simulink model "FOC_Simulate"  (R2023a)
settings: Solver=FixedStepDiscrete  StartTime=0.0  StopTime=2  FixedStep=1e-6  RelTol=1e-3
values from neighbouring files (symbols this model uses):
  amplitude_voltage = 12    [PMSM_default.m]
  pair_num = 4    [PMSM_default.m]
  speed_pid_d = 0.0    (= 0)    [PMSM_default.m]
  speed_pid_i = 10.0    (= 10)    [PMSM_default.m]
  speed_pid_integ_limit = 50.0    (= 50)    [PMSM_default.m]
  speed_pid_out_limit = 200.0    (= 200)    [PMSM_default.m]
  speed_pid_p = 50.0    (= 50)    [PMSM_default.m]
  svpwm_period = 1/1000    (= 0.001)    [PMSM_default.m]
  torque_Id_integ_limit = 10.0    (= 10)    [PMSM_default.m]
  torque_Id_out_limit = 100.0    (= 100)    [PMSM_default.m]
  torque_Id_pid_i = 5.0    (= 5)    [PMSM_default.m]
  torque_Id_pid_p = 75.0    (= 75)    [PMSM_default.m]
  torque_Iq_integ_limit = 20.0    (= 20)    [PMSM_default.m]
  torque_Iq_out_limit = 100.0    (= 100)    [PMSM_default.m]
  torque_Iq_pid_d = 0.0    (= 0)    [PMSM_default.m]
  torque_Iq_pid_i = 1.0    (= 1)    [PMSM_default.m]
  torque_Iq_pid_p = 1.0    (= 1)    [PMSM_default.m]
libraries: slpidlib x4, simulink x2, spsDCVoltageSourceLib x1, spsPermanentMagnetSynchronousMachineLib x1, spsTwoLevelConverterLib x1, sps_lib x1
settings Model: Creator=72698  LastModifiedBy=72698
settings SolverCC: AutoInsertRateTranBlk=on

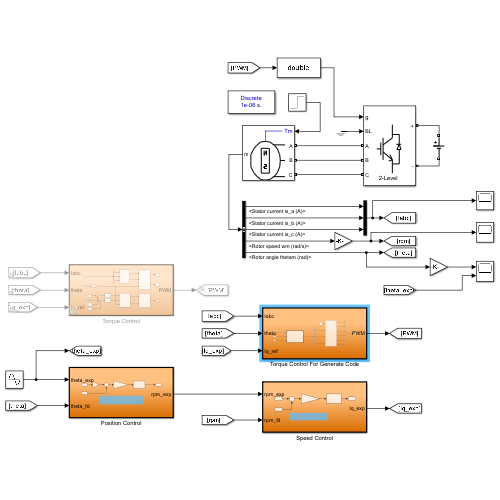
[thumbnail: Simulink's stored preview of the top-level diagram]
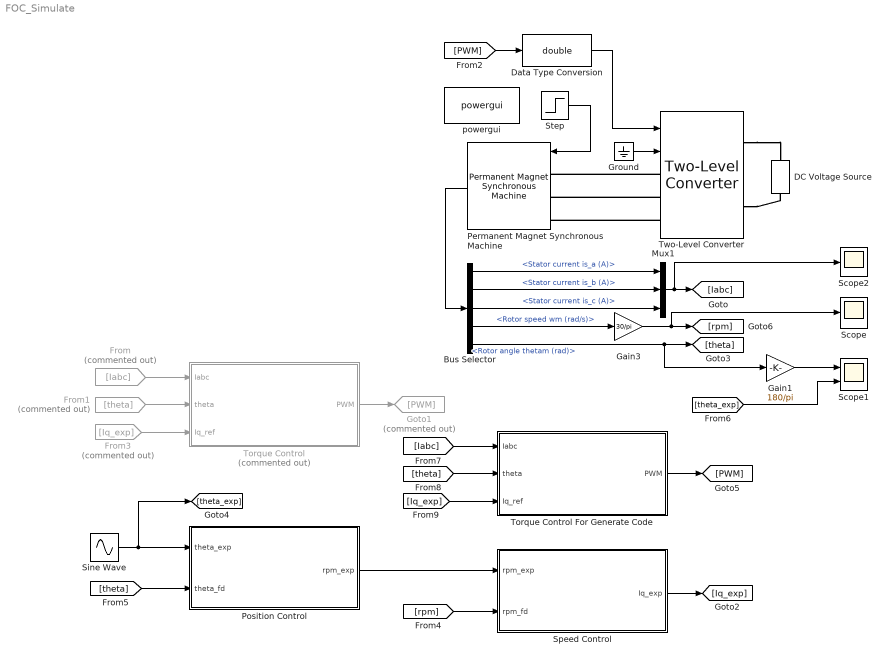
== system FOC_Simulate ==
  Bus Selector : BusSelector  OutputSignals=Stator current is_a (A),Stator current is_b (A),Stator current is_c (A),Rotor speed wm (rad/s),Rotor angle thetam (rad)
  DC Voltage Source : spsDCVoltageSourceLib/DC Voltage Source  Amplitude=amplitude_voltage  Measurements=None
  Data Type Conversion : DataTypeConversion  OutDataTypeStr=double  SaturateOnIntegerOverflow=off  RndMeth=Floor
  From : From  Commented=on  GotoTag=Iabc
  From1 : From  Commented=on  GotoTag=theta
  From3 : From  Commented=on  GotoTag=Iq_exp
  Gain1 : Gain  Gain=180/pi
  Gain3 : Gain  Gain=30/pi
  Goto1 : Goto  Commented=on  GotoTag=PWM
  Ground : Ground
  Mux1 : Mux  Inputs=3
  Permanent Magnet Synchronous Machine : spsPermanentMagnetSynchronousMachineLib/Permanent Magnet Synchronous Machine  NbPhases=3  FluxDistribution=Sinusoidal  RotorType=Round  MechanicalLoad=Torque Tm  PresetModel=No  ShowDetailedParameters=on  MeasurementBus=off  Resistance=0.0485  Inductance=8.5e-3  dqInductances=[8.5e-3,8.5e-3]  La=0.000395  MachineConstant=Flux linkage established by magnets (V.s)  Flux=0.1194  VoltageCst=86.6271  TorqueCst=0.7164  Flat=120  Mechanical=[0.0027 0.0004924 pair_num 0]  PolePairs=4  InitialConditions=[0,0, 0,0]  InitialConditions5ph=[0 0 0 0 0 0]  RefAngle=Aligned with phase A axis (original Park)  IterativeDiscreteModel=Trapezoidal non iterative  TsBlock=-1  TsPowergui=0
  Position Control : Subsystem  TreatAsAtomicUnit=on
  Scope : Scope
  Scope1 : Scope  NumInputPorts=2
  Scope2 : Scope
  Sine Wave : Sin  Amplitude=100  Frequency=10  SampleTime=0
  Speed Control : Subsystem  TreatAsAtomicUnit=on
  Step : Step  Time=0.2  After=10  SampleTime=0
  Torque Control : Subsystem  Commented=on  TreatAsAtomicUnit=on
  Torque Control For Generate Code : Subsystem  TreatAsAtomicUnit=on
  Two-Level Converter : spsTwoLevelConverterLib/Two-Level Converter  ModelType=Switching devices  Ron=1e-3  Rs=1e6  Cs=inf  Vforward=[0,0]  Ron_Diode=1e-3  Rs_Diode=1e6  Cs_Diode=inf  Vf_Diode=1e-3  Rs_CurrentSource=inf  Ron_ACsource=1e-3
      settings: LibrarySourceBlock=sps_lib/Power Electronics/Two-Level Converter
  powergui : sps_lib/powergui  Priority=1  SimulationMode=Discrete  SampleTime=1e-6  frequency=60  Iterations=50  frequencyindice=0  Pbase=100e6  ErrMax=1e-4  UnitsV=kV  UnitsW=MW  buscounter=0  FunctionMessages=off  echomessages=off  EnableUseOfTLC=off  CurrentSourceSwitches=off  DisableSnubberDevices=off  DisableRonSwitches=off  DisableVfSwitches=off  DisplayEquations=off  AutomaticDiscreteSolvers=off  SolverType=Tustin/Backward Euler (TBE)  Interpol=off  ExternalGateDelay=off  methode=off  Ts=100  x0status=blocks  SPID=on  SwTol=0  HookPort=off  NonlinearTolerance=1e-4  nMaxIteration=100  ContinueOnMaxIteration=off  RestoreLinks=warning  ResistiveCurrentMeasurement=off  Frange=[0:2:500]  Ylog=off  Xlog=on  ShowGrid=off  save=off  variable=ZData  structure=0  ZoomFFT=off  StartTime=0.0  cycles=1  DisplayStyle=1  fundamental=60  FreqAxis=off  MaxFrequency=1000  frequencyindicesteady=1  RmsSteady=1  display=off
  wires:
  Ground/1 -> Two-Level Converter/2
  Step/1 -> Permanent Magnet Synchronous Machine/1
  Permanent Magnet Synchronous Machine/1 -> Bus Selector/1
  Data Type Conversion/1 -> Two-Level Converter/1
  Bus Selector/4 -> Gain3/1  "<Rotor speed wm (rad/s)>"
  Bus Selector/5 -> Gain1/1, [theta]  "<Rotor angle thetam (rad)>"
  Bus Selector/1 -> Mux1/1  "<Stator current is_a (A)>"
  Bus Selector/2 -> Mux1/2  "<Stator current is_b (A)>"
  Bus Selector/3 -> Mux1/3  "<Stator current is_c (A)>"
  Mux1/1 -> Scope2/1, [Iabc]
  Gain3/1 -> Scope/1, [rpm]
  [PWM] -> Data Type Conversion/1
  [rpm] -> Speed Control/2(rpm_fd)
  Speed Control/1(Iq_exp) -> [Iq_exp]
  Gain1/1 -> Scope1/1
  Position Control/1(rpm_exp) -> Speed Control/1(rpm_exp)
  [theta] -> Position Control/2(theta_fd)
  Sine Wave/1 -> [theta_exp], Position Control/1(theta_exp)
  [theta_exp] -> Scope1/2
  Torque Control For Generate Code/1(PWM) -> [PWM]
  [theta] -> Torque Control For Generate Code/2(theta)
  [Iabc] -> Torque Control For Generate Code/1(Iabc)
  [Iq_exp] -> Torque Control For Generate Code/3(Iq_ref)
  Torque Control/1(PWM) -> Goto1/1
  From1/1 -> Torque Control/2(theta)
  From/1 -> Torque Control/1(Iabc)
  From3/1 -> Torque Control/3(Iq_ref)
  connections:
  Two-Level Converter/LConn1 -- Permanent Magnet Synchronous Machine/LConn1
  Two-Level Converter/LConn2 -- Permanent Magnet Synchronous Machine/LConn2
  Two-Level Converter/LConn3 -- Permanent Magnet Synchronous Machine/LConn3
  Two-Level Converter/RConn1 -- DC Voltage Source/RConn1
  Two-Level Converter/RConn2 -- DC Voltage Source/LConn1

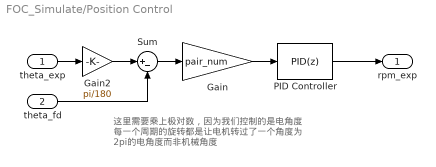
== system FOC_Simulate/Position Control ==
  note: 这里需要乘上极对数，因为我们控制的是电角度
      | 每一个周期的旋转都是让电机转过了一个角度为
      | 2pi的电角度而非机械角度
  theta_exp : Inport
  theta_fd : Inport  Port=2
  Gain : Gain  Gain=pair_num
  Gain2 : Gain  Gain=pi/180
  PID Controller : slpidlib/PID Controller  Controller=PID  Form=Parallel  TimeDomain=Discrete-time  UseExternalTs=off  SampleTime=-1  IntegratorMethod=Forward Euler  FilterMethod=Forward Euler  ControllerParametersSource=internal  P=95  I=0  UseKiTs=off  D=0  N=100  UseFilter=on  TunerSelectOption=Transfer Function Based (PID Tuner App)  InitialConditionSource=internal  InitialConditionForIntegrator=0  InitialConditionForFilter=0  DifferentiatorICPrevScaledInput=0  ExternalReset=none  TrackingMode=off  Kt=1  LimitOutput=on  SatLimitsSource=internal  UpperSaturationLimit=speed_pid_out_limit  LowerSaturationLimit=-speed_pid_out_limit  LinearizeAsGain=on  AntiWindupMode=none  Kb=1  LimitIntegrator=on  UpperIntegratorSaturationLimit=speed_pid_integ_limit  LowerIntegratorSaturationLimit=-speed_pid_integ_limit  POutMin=[]  POutMax=[]  IOutMin=[]  IOutMax=[]  DOutMin=[]  DOutMax=[]  NOutMin=[]  NOutMax=[]  SumOutMin=[]  SumOutMax=[]  SaturationOutMin=[]  SaturationOutMax=[]  PParamMin=[]  PParamMax=[]  IParamMin=[]  IParamMax=[]  DParamMin=[]  DParamMax=[]  NParamMin=[]  NParamMax=[]  KbParamMin=[]  KbParamMax=[]  KtParamMin=[]  KtParamMax=[]  KbOutMin=[]  KbOutMax=[]  KtOutMin=[]  KtOutMax=[]  IntegratorOutMin=[]  IntegratorOutMax=[]  FilterOutMin=[]  FilterOutMax=[]  SumI1OutMin=[]  SumI1OutMax=[]  SumI2OutMin=[]  SumI2OutMax=[]  SumI3OutMin=[]  SumI3OutMax=[]  SumI4OutMin=[]  SumI4OutMax=[]  SumDOutMin=[]  SumDOutMax=[]  DifferentiatorOutMin=[]  DifferentiatorOutMax=[]  FilterDiffOutCoefMin=[]  FilterDiffOutCoefMax=[]  ReciprocalOutMin=[]  ReciprocalOutMax=[]  SumDenOutMin=[]  SumDenOutMax=[]  SumNumOutMin=[]  SumNumOutMax=[]  DivideOutMin=[]  DivideOutMax=[]  UdiffTsProdOutMin=[]  UdiffTsProdOutMax=[]  NTsProdOutMin=[]  NTsProdOutMax=[]  UintegralTsProdOutMin=[]  UintegralTsProdOutMax=[]  UngainTsProdOutMin=[]  UngainTsProdOutMax=[]  ClampingZeroOutDataTypeStr=Inherit: Inherit via back propagation  ClampingZeroOutMin=[]  ClampingZeroOutMax=[]  FilterDenConstantOutDataTypeStr=Inherit: Inherit via back propagation  FilterDenConstantOutMin=[]  FilterDenConstantOutMax=[]  PCopyOutDataTypeStr=Inherit: Inherit via back propagation  PCopyOutMin=[]  PCopyOutMax=[]  NCopyOutDataTypeStr=Inherit: Inherit via back propagation  NCopyOutMin=[]  NCopyOutMax=[]  IntegratorContinuousStateAttributes=''  IntegratorStateMustResolveToSignalObject=off  IntegratorRTWStateStorageClass=Auto  FilterContinuousStateAttributes=''  FilterStateMustResolveToSignalObject=off  FilterRTWStateStorageClass=Auto  ParallelPVariant=InternalParameters  IdealPVariant=Disabled  IVariant=InternalParameters  DVariant=InternalParameters  IntegratorVariant=Discrete  SatVariant=Enabled  AWVariant=Passthrough  PCopyVariant=Disabled  TRVariant=Disabled  FdbkBlocksVariant=Forward  IdealPFdbkVariant=Disabled  SatFdbkVariant=Disabled  DerivativeFilterVariant=ForwardEulerFilter  NVariant=InternalParameters  NCopyVariant=Disabled  FilterICVariant=InternalICsFilter  IntegratorICVariant=InternalICs  ExternalResetVariant=Disabled  TRSumVariant=Passthrough  SumFdbkVariant=Disabled  SumVariant=Sum_PID  TsampFilterVariant=InternalTs  TsampNgainVariant=Passthrough  TsampIntegralVariant=Disabled_SignalSpec  ExternalSaturationOutDataTypeStr=Inherit: Same as second input
  Sum : Sum  Inputs=|+-
  rpm_exp : Outport
  wires:
  Gain/1 -> PID Controller/1
  Gain2/1 -> Sum/1
  theta_exp/1 -> Gain2/1
  Sum/1 -> Gain/1
  theta_fd/1 -> Sum/2
  PID Controller/1 -> rpm_exp/1

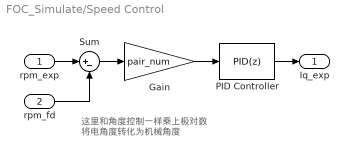
== system FOC_Simulate/Speed Control ==
  note: 这里和角度控制一样乘上极对数
      | 将电角度转化为机械角度
  rpm_exp : Inport
  rpm_fd : Inport  Port=2
  Gain : Gain  Gain=pair_num
  PID Controller : slpidlib/PID Controller  Controller=PID  Form=Parallel  TimeDomain=Discrete-time  UseExternalTs=off  SampleTime=-1  IntegratorMethod=Forward Euler  FilterMethod=Forward Euler  ControllerParametersSource=internal  P=speed_pid_p  I=speed_pid_i  UseKiTs=off  D=speed_pid_d  N=100  UseFilter=on  TunerSelectOption=Transfer Function Based (PID Tuner App)  InitialConditionSource=internal  InitialConditionForIntegrator=0  InitialConditionForFilter=0  DifferentiatorICPrevScaledInput=0  ExternalReset=none  TrackingMode=off  Kt=1  LimitOutput=on  SatLimitsSource=internal  UpperSaturationLimit=speed_pid_out_limit  LowerSaturationLimit=-speed_pid_out_limit  LinearizeAsGain=on  AntiWindupMode=none  Kb=1  LimitIntegrator=on  UpperIntegratorSaturationLimit=speed_pid_integ_limit  LowerIntegratorSaturationLimit=-speed_pid_integ_limit  POutMin=[]  POutMax=[]  IOutMin=[]  IOutMax=[]  DOutMin=[]  DOutMax=[]  NOutMin=[]  NOutMax=[]  SumOutMin=[]  SumOutMax=[]  SaturationOutMin=[]  SaturationOutMax=[]  PParamMin=[]  PParamMax=[]  IParamMin=[]  IParamMax=[]  DParamMin=[]  DParamMax=[]  NParamMin=[]  NParamMax=[]  KbParamMin=[]  KbParamMax=[]  KtParamMin=[]  KtParamMax=[]  KbOutMin=[]  KbOutMax=[]  KtOutMin=[]  KtOutMax=[]  IntegratorOutMin=[]  IntegratorOutMax=[]  FilterOutMin=[]  FilterOutMax=[]  SumI1OutMin=[]  SumI1OutMax=[]  SumI2OutMin=[]  SumI2OutMax=[]  SumI3OutMin=[]  SumI3OutMax=[]  SumI4OutMin=[]  SumI4OutMax=[]  SumDOutMin=[]  SumDOutMax=[]  DifferentiatorOutMin=[]  DifferentiatorOutMax=[]  FilterDiffOutCoefMin=[]  FilterDiffOutCoefMax=[]  ReciprocalOutMin=[]  ReciprocalOutMax=[]  SumDenOutMin=[]  SumDenOutMax=[]  SumNumOutMin=[]  SumNumOutMax=[]  DivideOutMin=[]  DivideOutMax=[]  UdiffTsProdOutMin=[]  UdiffTsProdOutMax=[]  NTsProdOutMin=[]  NTsProdOutMax=[]  UintegralTsProdOutMin=[]  UintegralTsProdOutMax=[]  UngainTsProdOutMin=[]  UngainTsProdOutMax=[]  ClampingZeroOutDataTypeStr=Inherit: Inherit via back propagation  ClampingZeroOutMin=[]  ClampingZeroOutMax=[]  FilterDenConstantOutDataTypeStr=Inherit: Inherit via back propagation  FilterDenConstantOutMin=[]  FilterDenConstantOutMax=[]  PCopyOutDataTypeStr=Inherit: Inherit via back propagation  PCopyOutMin=[]  PCopyOutMax=[]  NCopyOutDataTypeStr=Inherit: Inherit via back propagation  NCopyOutMin=[]  NCopyOutMax=[]  IntegratorContinuousStateAttributes=''  IntegratorStateMustResolveToSignalObject=off  IntegratorRTWStateStorageClass=Auto  FilterContinuousStateAttributes=''  FilterStateMustResolveToSignalObject=off  FilterRTWStateStorageClass=Auto  ParallelPVariant=InternalParameters  IdealPVariant=Disabled  IVariant=InternalParameters  DVariant=InternalParameters  IntegratorVariant=Discrete  SatVariant=Enabled  AWVariant=Passthrough  PCopyVariant=Disabled  TRVariant=Disabled  FdbkBlocksVariant=Forward  IdealPFdbkVariant=Disabled  SatFdbkVariant=Disabled  DerivativeFilterVariant=ForwardEulerFilter  NVariant=InternalParameters  NCopyVariant=Disabled  FilterICVariant=InternalICsFilter  IntegratorICVariant=InternalICs  ExternalResetVariant=Disabled  TRSumVariant=Passthrough  SumFdbkVariant=Disabled  SumVariant=Sum_PID  TsampFilterVariant=InternalTs  TsampNgainVariant=Passthrough  TsampIntegralVariant=Disabled_SignalSpec  ExternalSaturationOutDataTypeStr=Inherit: Same as second input
  Sum : Sum  Inputs=|+-
  Iq_exp : Outport
  wires:
  rpm_exp/1 -> Sum/1
  rpm_fd/1 -> Sum/2
  Sum/1 -> Gain/1
  PID Controller/1 -> Iq_exp/1
  Gain/1 -> PID Controller/1

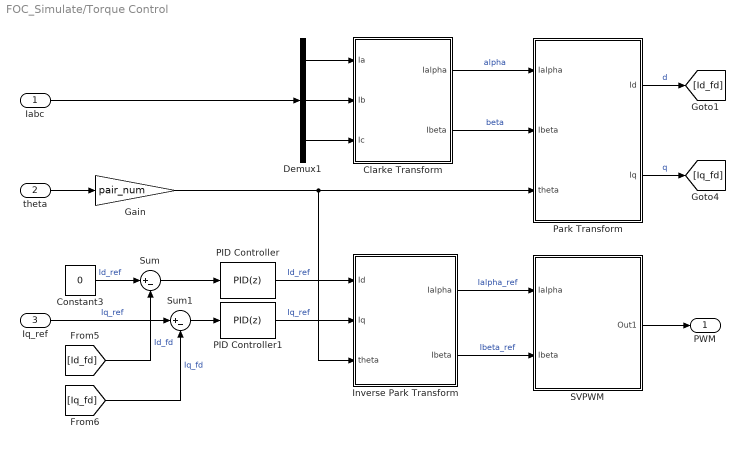
== system FOC_Simulate/Torque Control ==
  Iabc : Inport
  theta : Inport  Port=2
  Iq_ref : Inport  Port=3
  Clarke Transform : Subsystem  TreatAsAtomicUnit=on
  Constant3 : Constant  Value=0
  Demux1 : Demux  Outputs=3
  Gain : Gain  Gain=pair_num
  Inverse Park Transform : Subsystem  TreatAsAtomicUnit=on
  PID Controller : slpidlib/PID Controller  Controller=PID  Form=Parallel  TimeDomain=Discrete-time  UseExternalTs=off  SampleTime=-1  IntegratorMethod=Forward Euler  FilterMethod=Forward Euler  ControllerParametersSource=internal  P=torque_Id_pid_p  I=torque_Id_pid_i  UseKiTs=off  D=torque_Iq_pid_d  N=100  UseFilter=on  TunerSelectOption=Transfer Function Based (PID Tuner App)  InitialConditionSource=internal  InitialConditionForIntegrator=0  InitialConditionForFilter=0  DifferentiatorICPrevScaledInput=0  ExternalReset=none  TrackingMode=off  Kt=1  LimitOutput=on  SatLimitsSource=internal  UpperSaturationLimit=torque_Id_out_limit  LowerSaturationLimit=-torque_Id_out_limit  LinearizeAsGain=on  AntiWindupMode=none  Kb=1  LimitIntegrator=on  UpperIntegratorSaturationLimit=torque_Id_integ_limit  LowerIntegratorSaturationLimit=-torque_Id_integ_limit  POutMin=[]  POutMax=[]  IOutMin=[]  IOutMax=[]  DOutMin=[]  DOutMax=[]  NOutMin=[]  NOutMax=[]  SumOutMin=[]  SumOutMax=[]  SaturationOutMin=[]  SaturationOutMax=[]  PParamMin=[]  PParamMax=[]  IParamMin=[]  IParamMax=[]  DParamMin=[]  DParamMax=[]  NParamMin=[]  NParamMax=[]  KbParamMin=[]  KbParamMax=[]  KtParamMin=[]  KtParamMax=[]  KbOutMin=[]  KbOutMax=[]  KtOutMin=[]  KtOutMax=[]  IntegratorOutMin=[]  IntegratorOutMax=[]  FilterOutMin=[]  FilterOutMax=[]  SumI1OutMin=[]  SumI1OutMax=[]  SumI2OutMin=[]  SumI2OutMax=[]  SumI3OutMin=[]  SumI3OutMax=[]  SumI4OutMin=[]  SumI4OutMax=[]  SumDOutMin=[]  SumDOutMax=[]  DifferentiatorOutMin=[]  DifferentiatorOutMax=[]  FilterDiffOutCoefMin=[]  FilterDiffOutCoefMax=[]  ReciprocalOutMin=[]  ReciprocalOutMax=[]  SumDenOutMin=[]  SumDenOutMax=[]  SumNumOutMin=[]  SumNumOutMax=[]  DivideOutMin=[]  DivideOutMax=[]  UdiffTsProdOutMin=[]  UdiffTsProdOutMax=[]  NTsProdOutMin=[]  NTsProdOutMax=[]  UintegralTsProdOutMin=[]  UintegralTsProdOutMax=[]  UngainTsProdOutMin=[]  UngainTsProdOutMax=[]  ClampingZeroOutDataTypeStr=Inherit: Inherit via back propagation  ClampingZeroOutMin=[]  ClampingZeroOutMax=[]  FilterDenConstantOutDataTypeStr=Inherit: Inherit via back propagation  FilterDenConstantOutMin=[]  FilterDenConstantOutMax=[]  PCopyOutDataTypeStr=Inherit: Inherit via back propagation  PCopyOutMin=[]  PCopyOutMax=[]  NCopyOutDataTypeStr=Inherit: Inherit via back propagation  NCopyOutMin=[]  NCopyOutMax=[]  IntegratorContinuousStateAttributes=''  IntegratorStateMustResolveToSignalObject=off  IntegratorRTWStateStorageClass=Auto  FilterContinuousStateAttributes=''  FilterStateMustResolveToSignalObject=off  FilterRTWStateStorageClass=Auto  ParallelPVariant=InternalParameters  IdealPVariant=Disabled  IVariant=InternalParameters  DVariant=InternalParameters  IntegratorVariant=Discrete  SatVariant=Enabled  AWVariant=Passthrough  PCopyVariant=Disabled  TRVariant=Disabled  FdbkBlocksVariant=Forward  IdealPFdbkVariant=Disabled  SatFdbkVariant=Disabled  DerivativeFilterVariant=ForwardEulerFilter  NVariant=InternalParameters  NCopyVariant=Disabled  FilterICVariant=InternalICsFilter  IntegratorICVariant=InternalICs  ExternalResetVariant=Disabled  TRSumVariant=Passthrough  SumFdbkVariant=Disabled  SumVariant=Sum_PID  TsampFilterVariant=InternalTs  TsampNgainVariant=Passthrough  TsampIntegralVariant=Disabled_SignalSpec  ExternalSaturationOutDataTypeStr=Inherit: Same as second input
  PID Controller1 : slpidlib/PID Controller  Controller=PID  Form=Parallel  TimeDomain=Discrete-time  UseExternalTs=off  SampleTime=-1  IntegratorMethod=Forward Euler  FilterMethod=Forward Euler  ControllerParametersSource=internal  P=torque_Iq_pid_p  I=torque_Iq_pid_i  UseKiTs=off  D=torque_Iq_pid_d  N=100  UseFilter=on  TunerSelectOption=Transfer Function Based (PID Tuner App)  InitialConditionSource=internal  InitialConditionForIntegrator=0  InitialConditionForFilter=0  DifferentiatorICPrevScaledInput=0  ExternalReset=none  TrackingMode=off  Kt=1  LimitOutput=on  SatLimitsSource=internal  UpperSaturationLimit=torque_Iq_out_limit  LowerSaturationLimit=-torque_Iq_out_limit  LinearizeAsGain=on  AntiWindupMode=none  Kb=1  LimitIntegrator=on  UpperIntegratorSaturationLimit=torque_Iq_integ_limit  LowerIntegratorSaturationLimit=-torque_Iq_integ_limit  POutMin=[]  POutMax=[]  IOutMin=[]  IOutMax=[]  DOutMin=[]  DOutMax=[]  NOutMin=[]  NOutMax=[]  SumOutMin=[]  SumOutMax=[]  SaturationOutMin=[]  SaturationOutMax=[]  PParamMin=[]  PParamMax=[]  IParamMin=[]  IParamMax=[]  DParamMin=[]  DParamMax=[]  NParamMin=[]  NParamMax=[]  KbParamMin=[]  KbParamMax=[]  KtParamMin=[]  KtParamMax=[]  KbOutMin=[]  KbOutMax=[]  KtOutMin=[]  KtOutMax=[]  IntegratorOutMin=[]  IntegratorOutMax=[]  FilterOutMin=[]  FilterOutMax=[]  SumI1OutMin=[]  SumI1OutMax=[]  SumI2OutMin=[]  SumI2OutMax=[]  SumI3OutMin=[]  SumI3OutMax=[]  SumI4OutMin=[]  SumI4OutMax=[]  SumDOutMin=[]  SumDOutMax=[]  DifferentiatorOutMin=[]  DifferentiatorOutMax=[]  FilterDiffOutCoefMin=[]  FilterDiffOutCoefMax=[]  ReciprocalOutMin=[]  ReciprocalOutMax=[]  SumDenOutMin=[]  SumDenOutMax=[]  SumNumOutMin=[]  SumNumOutMax=[]  DivideOutMin=[]  DivideOutMax=[]  UdiffTsProdOutMin=[]  UdiffTsProdOutMax=[]  NTsProdOutMin=[]  NTsProdOutMax=[]  UintegralTsProdOutMin=[]  UintegralTsProdOutMax=[]  UngainTsProdOutMin=[]  UngainTsProdOutMax=[]  ClampingZeroOutDataTypeStr=Inherit: Inherit via back propagation  ClampingZeroOutMin=[]  ClampingZeroOutMax=[]  FilterDenConstantOutDataTypeStr=Inherit: Inherit via back propagation  FilterDenConstantOutMin=[]  FilterDenConstantOutMax=[]  PCopyOutDataTypeStr=Inherit: Inherit via back propagation  PCopyOutMin=[]  PCopyOutMax=[]  NCopyOutDataTypeStr=Inherit: Inherit via back propagation  NCopyOutMin=[]  NCopyOutMax=[]  IntegratorContinuousStateAttributes=''  IntegratorStateMustResolveToSignalObject=off  IntegratorRTWStateStorageClass=Auto  FilterContinuousStateAttributes=''  FilterStateMustResolveToSignalObject=off  FilterRTWStateStorageClass=Auto  ParallelPVariant=InternalParameters  IdealPVariant=Disabled  IVariant=InternalParameters  DVariant=InternalParameters  IntegratorVariant=Discrete  SatVariant=Enabled  AWVariant=Passthrough  PCopyVariant=Disabled  TRVariant=Disabled  FdbkBlocksVariant=Forward  IdealPFdbkVariant=Disabled  SatFdbkVariant=Disabled  DerivativeFilterVariant=ForwardEulerFilter  NVariant=InternalParameters  NCopyVariant=Disabled  FilterICVariant=InternalICsFilter  IntegratorICVariant=InternalICs  ExternalResetVariant=Disabled  TRSumVariant=Passthrough  SumFdbkVariant=Disabled  SumVariant=Sum_PID  TsampFilterVariant=InternalTs  TsampNgainVariant=Passthrough  TsampIntegralVariant=Disabled_SignalSpec  ExternalSaturationOutDataTypeStr=Inherit: Same as second input
  Park Transform : Subsystem  TreatAsAtomicUnit=on
  SVPWM : Subsystem  TreatAsAtomicUnit=on
  Sum : Sum  Inputs=|+-
  Sum1 : Sum  Inputs=|+-
  PWM : Outport
  wires:
  Park Transform/2(Iq) -> [Iq_fd]  "q"
  Iq_ref/1 -> Sum1/1  "Iq_ref"
  [Iq_fd] -> Sum1/2  "Iq_fd"
  [Id_fd] -> Sum/2  "Id_fd"
  Demux1/2 -> Clarke Transform/2(Ib)
  Clarke Transform/1(Ialpha) -> Park Transform/1(Ialpha)  "alpha"
  PID Controller1/1 -> Inverse Park Transform/2(Iq)  "Iq_ref"
  theta/1 -> Gain/1
  Inverse Park Transform/1(Ialpha) -> SVPWM/1(Ialpha)  "Ialpha_ref"
  SVPWM/1(Out1) -> PWM/1
  Inverse Park Transform/2(Ibeta) -> SVPWM/2(Ibeta)  "Ibeta_ref"
  Demux1/1 -> Clarke Transform/1(Ia)
  Demux1/3 -> Clarke Transform/3(Ic)
  PID Controller/1 -> Inverse Park Transform/1(Id)  "Id_ref"
  Sum1/1 -> PID Controller1/1
  Clarke Transform/2(Ibeta) -> Park Transform/2(Ibeta)  "beta"
  Park Transform/1(Id) -> [Id_fd]  "d"
  Sum/1 -> PID Controller/1
  Constant3/1 -> Sum/1  "Id_ref"
  Iabc/1 -> Demux1/1
  Gain/1 -> Park Transform/3(theta), Inverse Park Transform/3(theta)

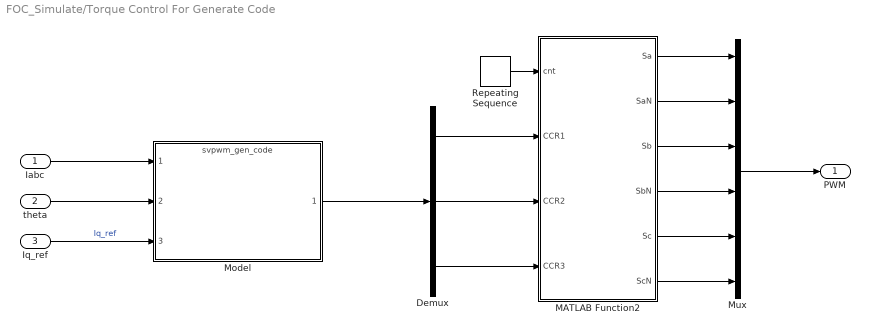
== system FOC_Simulate/Torque Control For Generate Code ==
  Iabc : Inport
  theta : Inport  Port=2
  Iq_ref : Inport  Port=3
  Demux : Demux  Outputs=3
  MATLAB Function2 : MATLAB Function  TreatAsAtomicUnit=on
  Model : ModelReference  ModelNameDialog=svpwm_gen_code.slx  SimulationMode=Normal  ModelReferenceVersion=1.1
  Mux : Mux  Inputs=6
  Repeating Sequence : simulink/Sources/Repeating Sequence  rep_seq_t=[0 svpwm_period/2 svpwm_period]  rep_seq_y=[0 svpwm_period/2 0]
  PWM : Outport
  wires:
  MATLAB Function2/4(SbN) -> Mux/4
  Repeating Sequence/1 -> MATLAB Function2/1(cnt)
  MATLAB Function2/5(Sc) -> Mux/5
  MATLAB Function2/6(ScN) -> Mux/6
  MATLAB Function2/3(Sb) -> Mux/3
  MATLAB Function2/1(Sa) -> Mux/1
  Demux/3 -> MATLAB Function2/4(CCR3)
  Demux/2 -> MATLAB Function2/3(CCR2)
  Demux/1 -> MATLAB Function2/2(CCR1)
  MATLAB Function2/2(SaN) -> Mux/2
  Iabc/1 -> Model/1
  theta/1 -> Model/2
  Iq_ref/1 -> Model/3  "Iq_ref"
  Model/1 -> Demux/1
  Mux/1 -> PWM/1

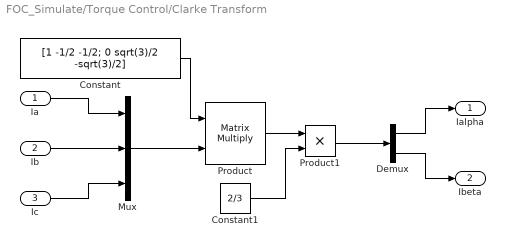
== system FOC_Simulate/Torque Control/Clarke Transform ==
  Ia : Inport
  Ib : Inport  Port=2
  Ic : Inport  Port=3
  Constant : Constant  Value=[1 -1/2 -1/2; 0 sqrt(3)/2 -sqrt(3)/2]
  Constant1 : Constant  Value=2/3
  Demux : Demux  Outputs=2
  Mux : Mux  Inputs=3
  Product : Product  Multiplication=Matrix(*)
  Product1 : Product
  Ialpha : Outport
  Ibeta : Outport  Port=2
  wires:
  Ib/1 -> Mux/2
  Ia/1 -> Mux/1
  Ic/1 -> Mux/3
  Mux/1 -> Product/2
  Constant/1 -> Product/1
  Demux/1 -> Ialpha/1
  Demux/2 -> Ibeta/1
  Product/1 -> Product1/1
  Product1/1 -> Demux/1
  Constant1/1 -> Product1/2

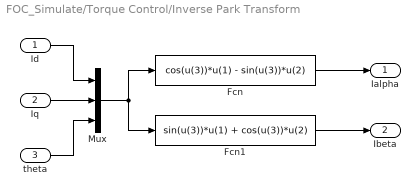
== system FOC_Simulate/Torque Control/Inverse Park Transform ==
  Id : Inport
  Iq : Inport  Port=2
  theta : Inport  Port=3
  Fcn : Fcn  Expr=cos(u(3))*u(1) - sin(u(3))*u(2)
  Fcn1 : Fcn  Expr=sin(u(3))*u(1) + cos(u(3))*u(2)
  Mux : Mux  Inputs=3
  Ialpha : Outport
  Ibeta : Outport  Port=2
  wires:
  Iq/1 -> Mux/2
  Id/1 -> Mux/1
  theta/1 -> Mux/3
  Mux/1 -> Fcn/1, Fcn1/1
  Fcn1/1 -> Ibeta/1
  Fcn/1 -> Ialpha/1

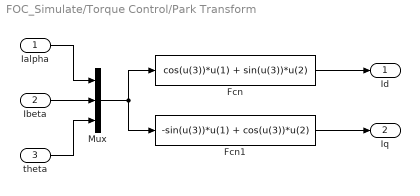
== system FOC_Simulate/Torque Control/Park Transform ==
  Ialpha : Inport
  Ibeta : Inport  Port=2
  theta : Inport  Port=3
  Fcn : Fcn  Expr=cos(u(3))*u(1) + sin(u(3))*u(2)
  Fcn1 : Fcn  Expr=-sin(u(3))*u(1) + cos(u(3))*u(2)
  Mux : Mux  Inputs=3
  Id : Outport
  Iq : Outport  Port=2
  wires:
  Ibeta/1 -> Mux/2
  Ialpha/1 -> Mux/1
  theta/1 -> Mux/3
  Mux/1 -> Fcn/1, Fcn1/1
  Fcn1/1 -> Iq/1
  Fcn/1 -> Id/1

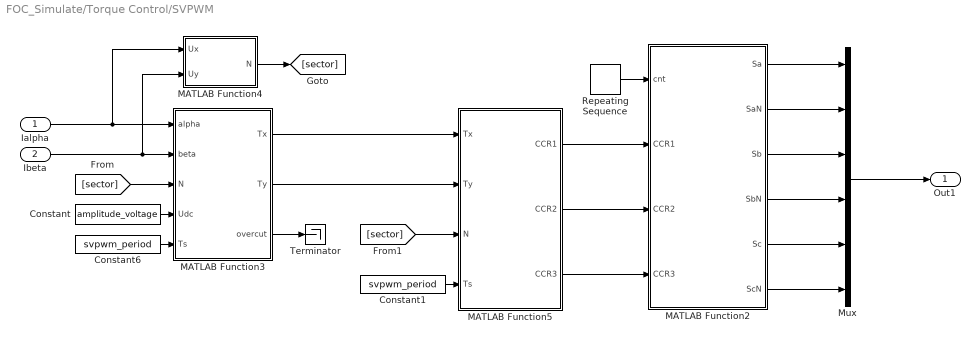
== system FOC_Simulate/Torque Control/SVPWM ==
  Ialpha : Inport
  Ibeta : Inport  Port=2
  Constant : Constant  Value=amplitude_voltage
  Constant1 : Constant  Value=svpwm_period
  Constant6 : Constant  Value=svpwm_period
  MATLAB Function2 : MATLAB Function  TreatAsAtomicUnit=on
  MATLAB Function3 : MATLAB Function  TreatAsAtomicUnit=on
  MATLAB Function4 : MATLAB Function  TreatAsAtomicUnit=on
  MATLAB Function5 : MATLAB Function  TreatAsAtomicUnit=on
  Mux : Mux  Inputs=6
  Repeating Sequence : simulink/Sources/Repeating Sequence  rep_seq_t=[0 svpwm_period/2 svpwm_period]  rep_seq_y=[0 svpwm_period/2 0]
  Terminator : Terminator
  Out1 : Outport
  wires:
  Ialpha/1 -> MATLAB Function4/1(Ux), MATLAB Function3/1(alpha)
  Ibeta/1 -> MATLAB Function4/2(Uy), MATLAB Function3/2(beta)
  Constant/1 -> MATLAB Function3/4(Udc)
  MATLAB Function3/1(Tx) -> MATLAB Function5/1(Tx)
  MATLAB Function3/2(Ty) -> MATLAB Function5/2(Ty)
  MATLAB Function5/1(CCR1) -> MATLAB Function2/2(CCR1)
  MATLAB Function5/2(CCR2) -> MATLAB Function2/3(CCR2)
  MATLAB Function5/3(CCR3) -> MATLAB Function2/4(CCR3)
  Repeating Sequence/1 -> MATLAB Function2/1(cnt)
  MATLAB Function2/1(Sa) -> Mux/1
  MATLAB Function2/2(SaN) -> Mux/2
  MATLAB Function2/3(Sb) -> Mux/3
  MATLAB Function2/4(SbN) -> Mux/4
  MATLAB Function2/5(Sc) -> Mux/5
  MATLAB Function2/6(ScN) -> Mux/6
  Constant1/1 -> MATLAB Function5/4(Ts)
  MATLAB Function4/1(N) -> [sector]
  [sector] -> MATLAB Function3/3(N)
  Constant6/1 -> MATLAB Function3/5(Ts)
  [sector] -> MATLAB Function5/3(N)
  MATLAB Function3/3(overcut) -> Terminator/1
  Mux/1 -> Out1/1

== matlab function FOC_Simulate/Torque Control/SVPWM/MATLAB Function4 ==
  data: Ux input; N output; Uy input
function N = fcn(Ux, Uy)
% 为了在单片机内快速判断扇区，因此要尽量规避三角函数操作，所以此处使用直线分隔的方式来判断当前扇区
if Uy > 0
    A = 0;
else
    A = 1;
end

if Uy - sqrt(3)*Ux > 0
    B = 0;
else
    B = 1;
end

if Uy + sqrt(3)*Ux > 0
    C = 0;
else
    C = 1;
end

dec = A*4 + B*2 + C;

switch dec
    case 2
        N = 1;
    case 0
        N = 2;
    case 1
        N = 3;
    case 5
        N = 4;
    case 7
        N= 5;
    otherwise
        N = 6;
end

== matlab function FOC_Simulate/Torque Control/SVPWM/MATLAB Function2 ==
  data: cnt input; Sa output; CCR1 input; CCR2 input; CCR3 input; SaN output; Sb output; SbN output; Sc output; ScN output
function [Sa, SaN, Sb, SbN, Sc, ScN] = fcn(cnt, CCR1, CCR2, CCR3)

if (cnt > CCR1)
    Sa = 1;
    SaN = 0;
else
    Sa = 0;
    SaN = 1;
end

if (cnt > CCR2)
    Sb = 1;
    SbN = 0;
else
    Sb = 0;
    SbN = 1;
end

if (cnt > CCR3)
    Sc = 1;
    ScN = 0;
else
    Sc = 0;
    ScN = 1;
end

== matlab function FOC_Simulate/Torque Control/SVPWM/MATLAB Function3 ==
  data: alpha input; beta input; N input; Tx output; Ty output; Udc input; Ts input; overcut output
function [Tx, Ty, overcut] = fcn(alpha, beta, N, Udc, Ts)
% 我们规定在旋转过程中，逆时针穿过该扇区时遇到的第一个基向量为v1，第二个基向量为v2
% m:调制比sqrt(3)*|Uref|/Udc
% |Uref|*sin(theta):合成矢量在alpha轴上的分量
% |Uref|*cos(theta):合成矢量在beta轴上的分量
value1 = (sqrt(3)/Udc) * Ts * beta;
value2 = (sqrt(3)/Udc) * Ts * (sqrt(3)*alpha + beta)* 0.5;
value3 = (sqrt(3)/Udc) * Ts * (-sqrt(3)*alpha + beta) * 0.5;

switch N
    case 1
        Tx = -value3;
        Ty = value1;
    case 2
        Tx = value3;
        Ty = value2;
    case 3
        Tx = value1;
        Ty = -value2;
    case 4
        Tx = -value1;
        Ty = value3;
    case 5
        Tx = -value2;
        Ty = -value3;
    otherwise
        Tx = value2;
        Ty = -value1;
end

if Tx+Ty > Ts
    overcut = 1;
    Tx_p = Tx; Ty_p = Ty;
    Tx = Ts * Tx_p / (Tx_p+Ty_p);
    Ty = Ts * Ty_p / (Tx_p+Ty_p);
else
    overcut = 0;
end

== matlab function FOC_Simulate/Torque Control For Generate Code/MATLAB Function2 ==
  data: cnt input; Sa output; CCR1 input; CCR2 input; CCR3 input; SaN output; Sb output; SbN output; Sc output; ScN output
function [Sa, SaN, Sb, SbN, Sc, ScN] = fcn(cnt, CCR1, CCR2, CCR3)

if (cnt > CCR1)
    Sa = 1;
    SaN = 0;
else
    Sa = 0;
    SaN = 1;
end

if (cnt > CCR2)
    Sb = 1;
    SbN = 0;
else
    Sb = 0;
    SbN = 1;
end

if (cnt > CCR3)
    Sc = 1;
    ScN = 0;
else
    Sc = 0;
    ScN = 1;
end

== matlab function FOC_Simulate/Torque Control/SVPWM/MATLAB Function5 ==
  data: Tx input; CCR1 output; Ty input; N input; CCR2 output; CCR3 output; Ts input
function [CCR1, CCR2, CCR3] = fcn(Tx, Ty, N, Ts)

value1 = (Ts-Tx-Ty) / 4;
value2 = value1 + Tx/2;
value3 = value2 + Ty/2;

switch N
    case 1
        CCR1 = value1;
        CCR2 = value2;
        CCR3 = value3;
    case 2
        CCR1 = value2;
        CCR2 = value1;
        CCR3 = value3;
    case 3
        CCR1 = value3;
        CCR2 = value1;
        CCR3 = value2;
    case 4
        CCR1 = value3;
        CCR2 = value2;
        CCR3 = value1;
    case 5
        CCR1 = value2;
        CCR2 = value3;
        CCR3 = value1;
    otherwise
        CCR1 = value1;
        CCR2 = value3;
        CCR3 = value2;
end
